simulink model "plcdemo_pid_feedforward"  (R2018a)
settings: Solver=ode8  StartTime=0.0  StopTime=200  FixedStep=1  RelTol=1e-5  EnableMultiTasking=on
undefined symbols (not defined in the file): A, B, C, DiscIntNeverNeededParam, FI, L
settings Model: Creator=The MathWorks, Inc.  LastModifiedBy=fugle
settings DataIOCC: LimitDataPoints=on  SaveFormat=Array
settings OptimizationCC: ExpressionDepthLimit=2147483647  LifeSpan=1
settings DebuggingCC: UnderspecifiedInitializationDetection=Classic  MergeDetectMultiDrivingBlocksExec=none  FcnCallInpInsideContextMsg=warning  StateNameClashWarn=warning  LibraryContextMissingDiagnostic=warning  SFUnexpectedBacktrackingDiag=warning  SFNoUnconditionalDefaultTransitionDiag=warning  SFExecutionAtInitializationDiag=none
settings HardwareCC: ProdBitPerPointer=32  ProdBitPerSizeT=32  ProdBitPerPtrDiffT=32  ProdLargestAtomicFloat=None  ProdIntDivRoundTo=Undefined  ProdEndianess=Unspecified  ProdWordSize=32  ProdHWDeviceType=32-bit Generic
settings ModelReferenceCC: PropagateSignalLabelsOutOfModel=off
settings SFSimCC: MATLABDynamicMemAlloc=off
settings RTWCC: SystemTargetFile=ert.tlc  TemplateMakefile=ert_default_tmf
settings CodeAppCC: IgnoreCustomStorageClasses=off  CustomSymbolStrType=$N$R$M  StateflowObjectComments=on  InternalIdentifier=Classic
settings ERTTargetCC: MultiwordLength=2048  GenerateSampleERTMain=on  ERTCustomFileTemplate=example_file_process.tlc  ConvertIfToSwitch=off  SuppressUnreachableDefaultCases=off
settings ConfigComp: CovMetricSettings=dw  CovHtmlReporting=on  CovSaveCumulativeToWorkspaceVar=on  CovSaveSingleToWorkspaceVar=on  CovExternalEMLEnable=off  PLC_OutputDir=./plcsrc  PLC_RTWShowEliminatedStatement=on  PLC_TargetIDE=codesys23  PLC_GenerateReport=off  PLC_LaunchReport=off

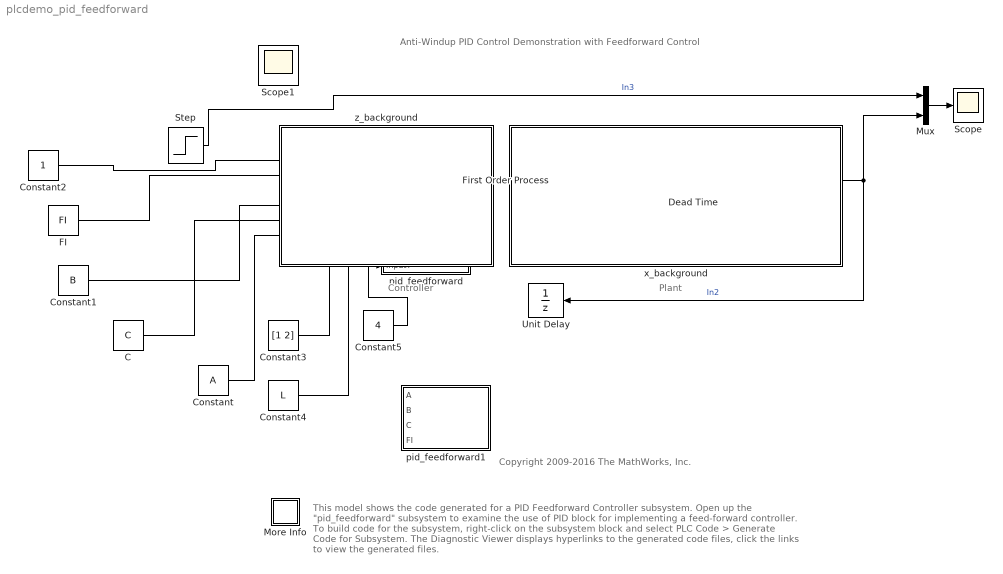
== system plcdemo_pid_feedforward ==
  note: Anti-Windup PID Control Demonstration
      | with Feedforward Control
  note: Copyright 2009-2016 The MathWorks, Inc.
  note: This model shows the code generated for a PID Feedforward Controller subsystem.
      | Open up the "pid_feedforward" subsystem to examine the use of PID block for implementing
      | a feed-forward controller.
      |
      | To build code for the subsystem, right-click on the subsystem block and
      | select PLC Code > Generate Code for Subsystem.
      |
      | The Diagnostic Viewer displays hyperlinks to the generated code files, click the links to view the generated files.
  note: Controller
  note: Plant
  C : Constant  Value=C  VectorParams1D=off
  Constant : Constant  Value=A  VectorParams1D=off
  Constant1 : Constant  Value=B  VectorParams1D=off
  Constant2 : Constant  VectorParams1D=off
  Constant3 : Constant  Value=[1 2]  VectorParams1D=off
  Constant4 : Constant  Value=L  VectorParams1D=off
  Constant5 : Constant  Value=4  VectorParams1D=off
  Dead Time : TransportDelay  DelayTime=2  BufferSize=2048
  FI : Constant  Value=FI
  First Order Process : TransferFcn  Numerator=1  Denominator=[10 1]
  More Info : Subsystem
      settings: OpenFcn=showdemo('sldemo_antiwindup')
      mask Display: disp('?')
  Mux : Mux  Inputs=2
  Scope : Scope
  Step : Step  Time=80  Before=10  After=5  SampleTime=0
  Unit Delay : UnitDelay  SampleTime=-1
  pid_feedforward : Subsystem  TreatAsAtomicUnit=on
  pid_feedforward1 : Subsystem  TreatAsAtomicUnit=on
  x_background : Subsystem
      mask Display: disp('')
  z_background : Subsystem  TreatAsAtomicUnit=on
      mask Display: disp('')
  Scope1 : Scope
  wires:
  First Order Process/1 -> Dead Time/1
  Step/1 -> Mux/1  "In3"
  Mux/1 -> Scope/1
  Dead Time/1 -> Unit Delay/1, Mux/2  "In2"
  FI/1 -> pid_feedforward/2(FI)
  Constant2/1 -> pid_feedforward/1(Ref)
  Constant3/1 -> pid_feedforward/3(F)
  Constant1/1 -> pid_feedforward/4(B)
  C/1 -> pid_feedforward/5(C)
  Constant/1 -> pid_feedforward/6(A)
  Constant4/1 -> pid_feedforward/7(L)
  Constant5/1 -> pid_feedforward/8(InputY)

== system plcdemo_pid_feedforward/More Info ==

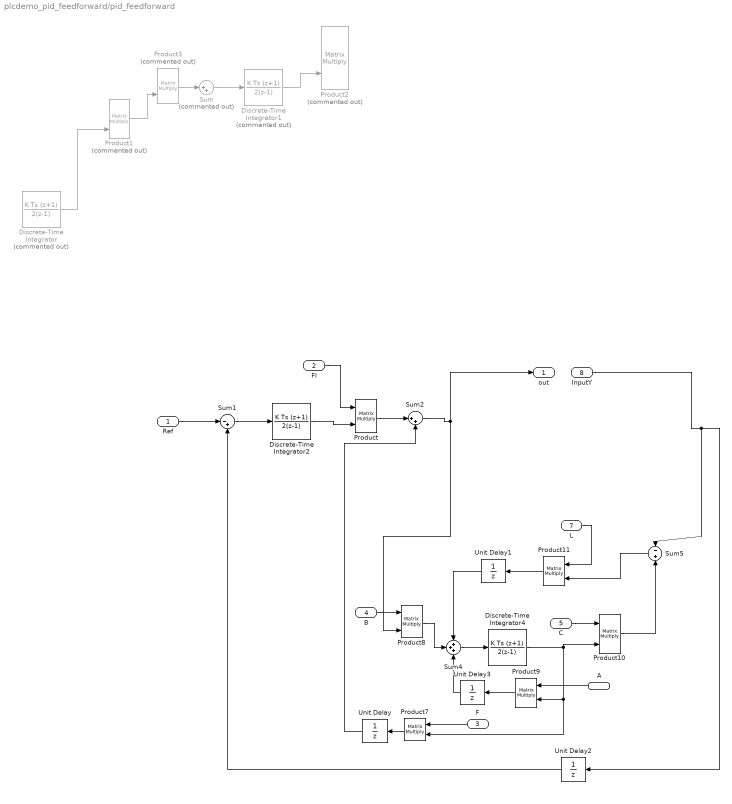
== system plcdemo_pid_feedforward/pid_feedforward ==
  Ref : Inport
  FI : Inport  Port=2
  F : Inport  Port=3
  B : Inport  Port=4
  C : Inport  Port=5
  A : Inport  Port=6
  L : Inport  Port=7
  InputY : Inport  Port=8
  Discrete-Time Integrator : DiscreteIntegrator  Commented=on  IntegratorMethod=Integration: Trapezoidal  SampleTime=-1  ICPrevOutput=DiscIntNeverNeededParam  ICPrevScaledInput=DiscIntNeverNeededParam
  Discrete-Time Integrator1 : DiscreteIntegrator  Commented=on  IntegratorMethod=Integration: Trapezoidal  SampleTime=-1  ICPrevOutput=DiscIntNeverNeededParam  ICPrevScaledInput=DiscIntNeverNeededParam
  Discrete-Time Integrator2 : DiscreteIntegrator  IntegratorMethod=Integration: Trapezoidal  SampleTime=-1  ICPrevOutput=DiscIntNeverNeededParam  ICPrevScaledInput=DiscIntNeverNeededParam
  Discrete-Time Integrator4 : DiscreteIntegrator  IntegratorMethod=Integration: Trapezoidal  SampleTime=-1  ICPrevOutput=DiscIntNeverNeededParam  ICPrevScaledInput=DiscIntNeverNeededParam
  Product{,7..11} (6 alike) : Product  Multiplication=Matrix(*)
  Product1 : Product  Commented=on  Multiplication=Matrix(*)
  Product2 : Product  Commented=on  Multiplication=Matrix(*)
  Product3 : Product  Commented=on  Multiplication=Matrix(*)
  Sum : Sum  Commented=on  Inputs=|++
  Sum1 : Sum  Inputs=|-+
  Sum2 : Sum  Inputs=|++
  Sum4 : Sum  Inputs=+++
  Sum5 : Sum  Inputs=-+
  Unit Delay{,1..3} (4 alike) : UnitDelay  SampleTime=-1
  out : Outport
  wires:
  Discrete-Time Integrator/1 -> Product1/2
  Product1/1 -> Product3/2
  Discrete-Time Integrator1/1 -> Product2/2
  Product3/1 -> Sum/1
  Sum/1 -> Discrete-Time Integrator1/1
  Ref/1 -> Sum1/1
  Sum1/1 -> Discrete-Time Integrator2/1
  Product/1 -> Sum2/1
  InputY/1 -> Sum5/1, Unit Delay2/1
  Product7/1 -> Unit Delay/1
  F/1 -> Product7/1
  Discrete-Time Integrator2/1 -> Product/2
  FI/1 -> Product/1
  Unit Delay/1 -> Sum2/2
  Unit Delay2/1 -> Sum1/2
  C/1 -> Product10/1
  B/1 -> Product8/1
  Product8/1 -> Sum4/2
  Sum2/1 -> out/1, Product8/2
  Product10/1 -> Sum5/2
  A/1 -> Product9/1
  Product9/1 -> Unit Delay3/1
  Discrete-Time Integrator4/1 -> Product10/2, Product9/2, Product7/2
  Unit Delay3/1 -> Sum4/3
  Sum4/1 -> Discrete-Time Integrator4/1
  L/1 -> Product11/1
  Sum5/1 -> Product11/2
  Product11/1 -> Unit Delay1/1
  Unit Delay1/1 -> Sum4/1

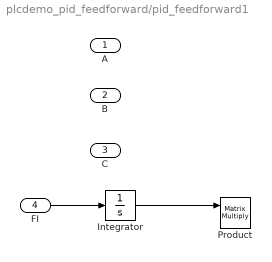
== system plcdemo_pid_feedforward/pid_feedforward1 ==
  A : Inport
  B : Inport  Port=2
  C : Inport  Port=3
  FI : Inport  Port=4
  Integrator : Integrator
  Product : Product  Multiplication=Matrix(*)
  wires:
  FI/1 -> Integrator/1
  Integrator/1 -> Product/1

== system plcdemo_pid_feedforward/x_background ==

== system plcdemo_pid_feedforward/z_background ==
